simulink model "sim25"  (R2013a)
settings: Solver=ode45  StartTime=0.0  StopTime=30  MaxStep=0.001  RelTol=1e-3
settings Model: Creator=hadisystem  LastModifiedBy=hadisystem

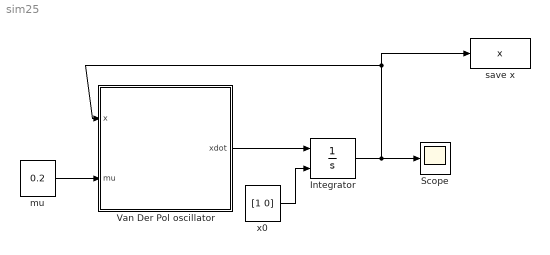
== system sim25 ==
  Integrator : Integrator  InitialConditionSource=external  InitialCondition=1
  Scope : Scope
  Van Der Pol oscillator : MATLAB Function  TreatAsAtomicUnit=on
  mu : Constant  Value=0.2
  "save x " : ToWorkspace  VariableName=x  SampleTime=-1  SaveFormat=Timeseries
  x0 : Constant  Value=[1 0]
  wires:
  mu/1 -> Van Der Pol oscillator/2(mu)
  Van Der Pol oscillator/1(xdot) -> Integrator/1
  Integrator/1 -> "save x "/1, Van Der Pol oscillator/1(x), Scope/1
  x0/1 -> Integrator/2

== matlab function sim25/Van Der Pol oscillator ==
  data: x input; xdot output; mu input
function xdot = fcn(x,mu)
xdot = [x(2)
    mu*(1-x(1)^2)*x(2)-x(1)];

end
